simulink model "Demonstration1_2024b"  (R2024b)
settings: Solver=ode15s  StartTime=0.0  StopTime=10  RelTol=1e-4
InitFcn:
  | clear all;
  | 
  | % Bauteilgrößen
  | R = 1e3;
  | L = 10e-3;
  | C1 = 100e-9;
  | C2 = 1e-6;
  | 
  | % weitere physikalische Größen
  | k  = 1.380649e-23;
  | e  = 1.602176634e-19;
  | T_C = 25;
  | T_K = 273.15;
  | T = T_C + T_K;
  | UT = k*T/e;
  | IS = 10e-9;
  | 
  | % U0 allgemein
  | U0 = 12;
  | 
  | % I0 für Regelstrecke (1. Fall)
  | I0_1 = 1e-3;
  | 
  | % I0 für Regelstrecke (2. Fall)
  | I0_2 = 3e-3;
  | 
  | % I0 für Regelstrecke (3. Fall)
  | I0_3 = 6e-3;
  | 
  | % I0 für lineare Zustandsrückführung
  | I0_ZRF = 10e-3;
  | 
  | % Berechnung von U2 in der GGL
  | U2_bar = -UT*log(1e8*I0_ZRF);
  | 
  | % Vorgabe der Eigenwerte
  | eigenvalues_ZRF = [-2-2i; -2+2i; -10];
  | 
  | % Jacobi-Matrizen an der GGL
  | A_ZRF = [0 IS/(C1*UT)*exp(-U2_bar/UT) 1/C1;
  |      	 0 0 1/C2;
  |          -1/L -1/L -R/L];
  | B_ZRF = [0, 0;
  |          0, -1/C2;
  |          1/L, 0];
  | 
  | % Reglermatrix für lineare ZRF
  | G_ZRF = place(A_ZRF,B_ZRF,eigenvalues_ZRF);
settings Model: Creator=richa  LastModifiedBy=richa
settings ConfigComp: CovBoundaryAbsTol=1.0e-5

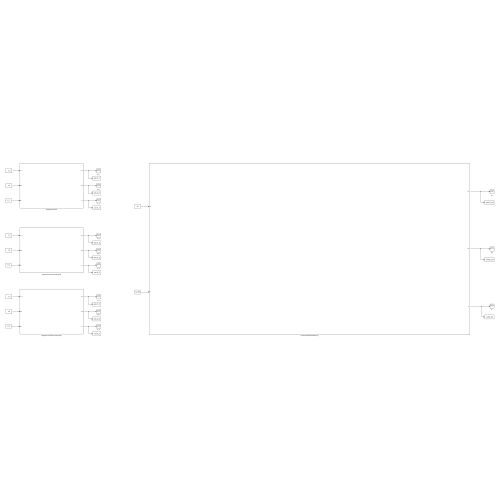
[thumbnail: Simulink's stored preview of the top-level diagram]
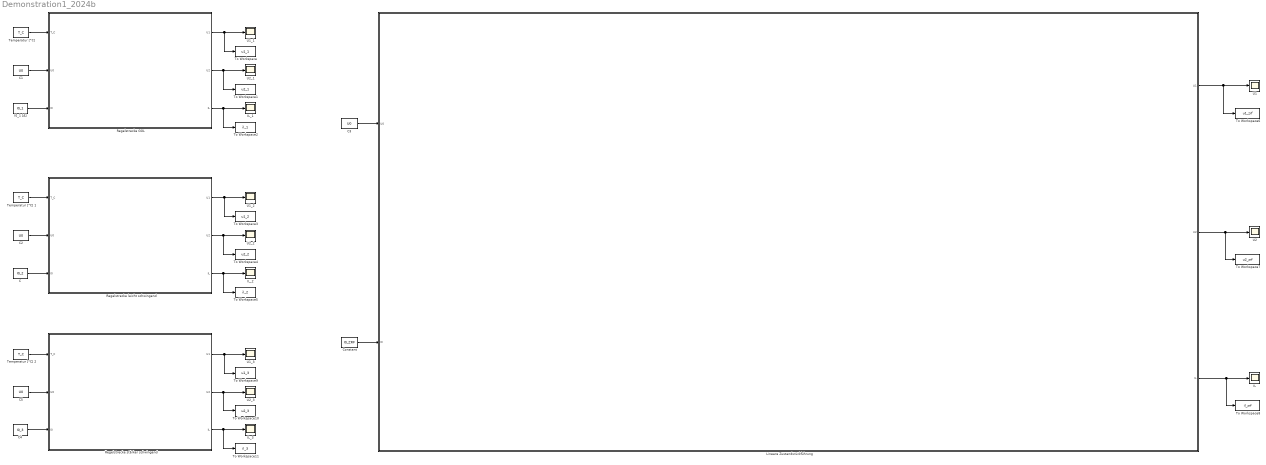
== system Demonstration1_2024b ==
  C : Constant  Value=I0_2
  C{1..3,5} (4 alike) : Constant  Value=U0
  C4 : Constant  Value=I0_3
  Constant : Constant  Value=I0_ZRF
  I0_1 [A] : Constant  Value=I0_1
  IL : Scope
  IL_1 : Scope
  IL_2 : Scope
  IL_3 : Scope
  Lineare Zustandsrückführung : Subsystem
  Regelstrecke GGL : Subsystem
  Regelstrecke leicht schwingend : Subsystem
  Regelstrecke stärker schwingend : Subsystem
  "Temperatur [°C] " : Constant  Value=T_C
  Temperatur [°C] 1 : Constant  Value=T_C
  Temperatur [°C] 2 : Constant  Value=T_C
  To Workspace : ToWorkspace  VariableName=u1_1  SaveFormat=Structure With Time  SampleTime=-1
  To Workspace1 : ToWorkspace  VariableName=u2_1  SaveFormat=Structure With Time  SampleTime=-1
  To Workspace10 : ToWorkspace  VariableName=u2_3  SaveFormat=Structure With Time  SampleTime=-1
  To Workspace11 : ToWorkspace  VariableName=il_3  SaveFormat=Structure With Time  SampleTime=-1
  To Workspace2 : ToWorkspace  VariableName=il_1  SaveFormat=Structure With Time  SampleTime=-1
  To Workspace3 : ToWorkspace  VariableName=u1_2  SaveFormat=Structure With Time  SampleTime=-1
  To Workspace4 : ToWorkspace  VariableName=u2_2  SaveFormat=Structure With Time  SampleTime=-1
  To Workspace5 : ToWorkspace  VariableName=il_2  SaveFormat=Structure With Time  SampleTime=-1
  To Workspace6 : ToWorkspace  VariableName=u1_zrf  SaveFormat=Structure With Time  SampleTime=-1
  To Workspace7 : ToWorkspace  VariableName=u2_zrf  SaveFormat=Structure With Time  SampleTime=-1
  To Workspace8 : ToWorkspace  VariableName=il_zrf  SaveFormat=Structure With Time  SampleTime=-1
  To Workspace9 : ToWorkspace  VariableName=u1_3  SaveFormat=Structure With Time  SampleTime=-1
  U1 : Scope
  U1_1 : Scope
  U1_2 : Scope
  U1_3 : Scope
  U2 : Scope
  U2_1 : Scope
  U2_2 : Scope
  U2_3 : Scope
  wires:
  "Temperatur [°C] "/1 -> Regelstrecke GGL/1(T_C)
  Regelstrecke GGL/1(U1) -> U1_1/1, To Workspace/1
  Regelstrecke GGL/2(U2) -> U2_1/1, To Workspace1/1
  Regelstrecke GGL/3(IL) -> IL_1/1, To Workspace2/1
  I0_1 [A]/1 -> Regelstrecke GGL/3(I0)
  C1/1 -> Regelstrecke GGL/2(U0)
  C/1 -> Regelstrecke leicht schwingend/3(I0)
  Regelstrecke leicht schwingend/3(IL) -> IL_2/1, To Workspace5/1
  Regelstrecke leicht schwingend/2(U2) -> U2_2/1, To Workspace4/1
  Regelstrecke leicht schwingend/1(U1) -> U1_2/1, To Workspace3/1
  Lineare Zustandsrückführung/3(IL) -> To Workspace8/1, IL/1
  Lineare Zustandsrückführung/1(U1) -> To Workspace6/1, U1/1
  Lineare Zustandsrückführung/2(U2) -> To Workspace7/1, U2/1
  Constant/1 -> Lineare Zustandsrückführung/2(I0)
  Temperatur [°C] 1/1 -> Regelstrecke leicht schwingend/1(T_C)
  C2/1 -> Regelstrecke leicht schwingend/2(U0)
  C3/1 -> Lineare Zustandsrückführung/1(U0)
  C4/1 -> Regelstrecke stärker schwingend/3(I0)
  C5/1 -> Regelstrecke stärker schwingend/2(U0)
  Regelstrecke stärker schwingend/2(U2) -> U2_3/1, To Workspace10/1
  Regelstrecke stärker schwingend/1(U1) -> U1_3/1, To Workspace9/1
  Regelstrecke stärker schwingend/3(IL) -> IL_3/1, To Workspace11/1
  Temperatur [°C] 2/1 -> Regelstrecke stärker schwingend/1(T_C)

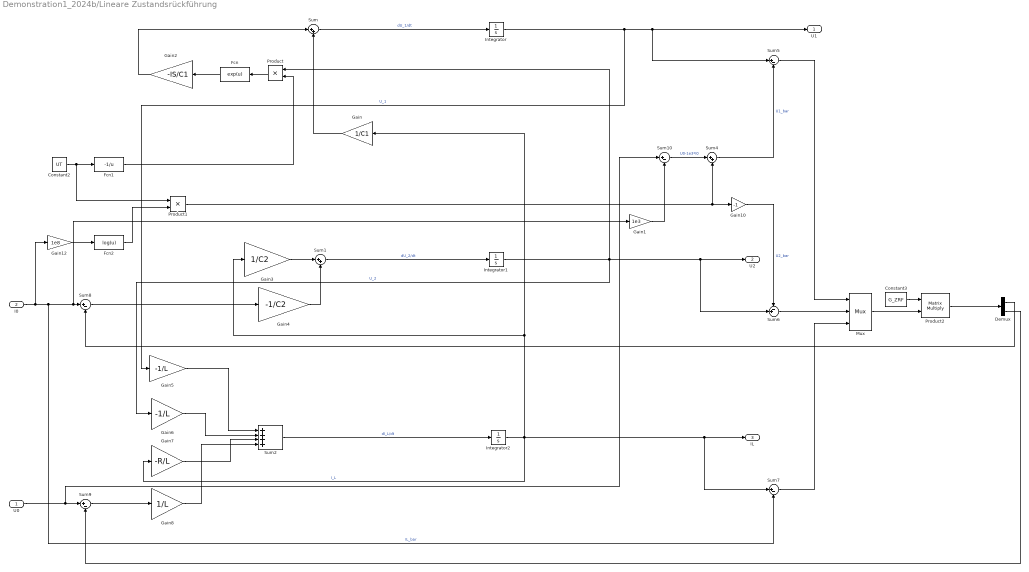
== system Demonstration1_2024b/Lineare Zustandsrückführung ==
  U0 : Inport
  I0 : Inport  Port=2
  Constant2 : Constant  Value=UT
  Constant3 : Constant  Value=G_ZRF
  Demux : Demux  Outputs=2
  Fcn : Fcn  Expr=exp(u)
  Fcn1 : Fcn  Expr=-1/u
  Fcn2 : Fcn  Expr=log(u)
  Gain : Gain  Gain=1/C1
  Gain1 : Gain  Gain=1e3
  Gain10 : Gain  Gain=-1
  Gain12 : Gain  Gain=1e8
  Gain2 : Gain  Gain=-IS/C1
  Gain3 : Gain  Gain=1/C2
  Gain4 : Gain  Gain=-1/C2
  Gain5 : Gain  Gain=-1/L
  Gain6 : Gain  Gain=-1/L
  Gain7 : Gain  Gain=-R/L
  Gain8 : Gain  Gain=1/L
  Integrator : Integrator
  Integrator1 : Integrator
  Integrator2 : Integrator
  Mux : Mux  Inputs=3
  Product : Product
  Product1 : Product
  Product2 : Product  Multiplication=Matrix(*)
  Sum : Sum  Inputs=|++
  Sum1 : Sum  Inputs=|++
  Sum{5,7..10} (5 alike) : Sum  Inputs=|+-
  Sum2 : Sum  Inputs=++++
  Sum4 : Sum  Inputs=|++
  Sum6 : Sum  Inputs=-+|
  U1 : Outport
  U2 : Outport  Port=2
  IL : Outport  Port=3
  wires:
  Integrator/1 -> U1/1, Sum5/1, Gain5/1  "U_1"
  Integrator2/1 -> Gain/1, Gain3/1, Gain7/1, IL/1, Sum7/1  "I_L"
  Gain4/1 -> Sum1/2
  Product/1 -> Fcn/1
  Constant2/1 -> Product1/1, Fcn1/1
  Gain/1 -> Sum/2
  Integrator1/1 -> U2/1, Sum6/2, Product/1, Gain6/1  "U_2"
  Gain10/1 -> Sum6/1  "U2_bar"
  Gain8/1 -> Sum2/4
  Gain3/1 -> Sum1/1
  I0/1 -> Gain12/1, Gain1/1, Sum8/1, Sum7/2  "IL_bar"
  Sum/1 -> Integrator/1  "dU_1/dt"
  Sum5/1 -> Mux/1
  Fcn1/1 -> Product/2
  Sum6/1 -> Mux/2
  Demux/2 -> Sum9/2
  Gain2/1 -> Sum/1
  Gain5/1 -> Sum2/1
  Sum8/1 -> Gain4/1
  Sum2/1 -> Integrator2/1  "dI_L/dt"
  Gain6/1 -> Sum2/2
  Sum4/1 -> Sum5/2  "U1_bar"
  Mux/1 -> Product2/2
  Sum10/1 -> Sum4/1  "U0-1e3*I0"
  Sum9/1 -> Gain8/1
  Product1/1 -> Gain10/1, Sum4/2
  Demux/1 -> Sum8/2
  Gain7/1 -> Sum2/3
  Fcn/1 -> Gain2/1
  Sum1/1 -> Integrator1/1  "dU_2/dt"
  Sum7/1 -> Mux/3
  Gain12/1 -> Fcn2/1
  Fcn2/1 -> Product1/2
  Gain1/1 -> Sum10/2
  Product2/1 -> Demux/1
  Constant3/1 -> Product2/1
  U0/1 -> Sum9/1, Sum10/1

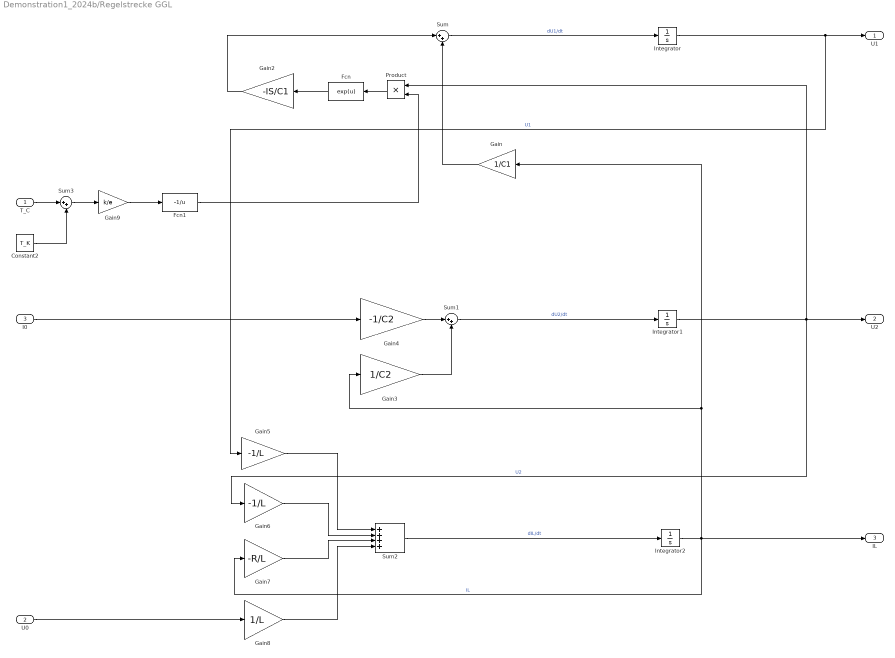
== system Demonstration1_2024b/Regelstrecke GGL ==
  T_C : Inport
  U0 : Inport  Port=2
  I0 : Inport  Port=3
  Constant2 : Constant  Value=T_K
  Fcn : Fcn  Expr=exp(u)
  Fcn1 : Fcn  Expr=-1/u
  Gain : Gain  Gain=1/C1
  Gain2 : Gain  Gain=-IS/C1
  Gain3 : Gain  Gain=1/C2
  Gain4 : Gain  Gain=-1/C2
  Gain5 : Gain  Gain=-1/L
  Gain6 : Gain  Gain=-1/L
  Gain7 : Gain  Gain=-R/L
  Gain8 : Gain  Gain=1/L
  Gain9 : Gain  Gain=k/e
  Integrator : Integrator
  Integrator1 : Integrator
  Integrator2 : Integrator
  Product : Product
  Sum : Sum  Inputs=|++
  Sum1 : Sum  Inputs=|++
  Sum2 : Sum  Inputs=++++
  Sum3 : Sum  Inputs=|++
  U1 : Outport
  U2 : Outport  Port=2
  IL : Outport  Port=3
  wires:
  Sum/1 -> Integrator/1  "dU1/dt"
  Integrator/1 -> U1/1, Gain5/1  "U1"
  Sum3/1 -> Gain9/1
  Gain2/1 -> Sum/1
  Gain8/1 -> Sum2/4
  Fcn1/1 -> Product/2
  Gain/1 -> Sum/2
  Gain9/1 -> Fcn1/1
  Gain5/1 -> Sum2/1
  I0/1 -> Gain4/1
  Gain7/1 -> Sum2/3
  U0/1 -> Gain8/1
  Sum1/1 -> Integrator1/1  "dU2/dt"
  Gain6/1 -> Sum2/2
  Integrator2/1 -> IL/1, Gain3/1, Gain/1, Gain7/1  "IL"
  Sum2/1 -> Integrator2/1  "dIL/dt"
  Gain4/1 -> Sum1/1
  Integrator1/1 -> U2/1, Product/1, Gain6/1  "U2"
  Constant2/1 -> Sum3/2
  Product/1 -> Fcn/1
  Fcn/1 -> Gain2/1
  Gain3/1 -> Sum1/2
  T_C/1 -> Sum3/1

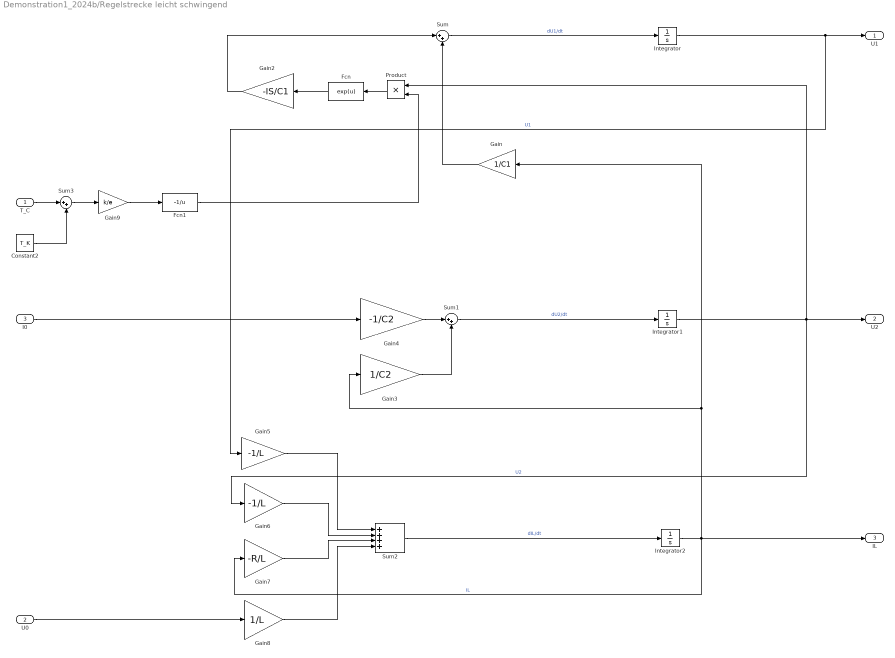
== system Demonstration1_2024b/Regelstrecke leicht schwingend ==
  T_C : Inport
  U0 : Inport  Port=2
  I0 : Inport  Port=3
  Constant2 : Constant  Value=T_K
  Fcn : Fcn  Expr=exp(u)
  Fcn1 : Fcn  Expr=-1/u
  Gain : Gain  Gain=1/C1
  Gain2 : Gain  Gain=-IS/C1
  Gain3 : Gain  Gain=1/C2
  Gain4 : Gain  Gain=-1/C2
  Gain5 : Gain  Gain=-1/L
  Gain6 : Gain  Gain=-1/L
  Gain7 : Gain  Gain=-R/L
  Gain8 : Gain  Gain=1/L
  Gain9 : Gain  Gain=k/e
  Integrator : Integrator
  Integrator1 : Integrator
  Integrator2 : Integrator
  Product : Product
  Sum : Sum  Inputs=|++
  Sum1 : Sum  Inputs=|++
  Sum2 : Sum  Inputs=++++
  Sum3 : Sum  Inputs=|++
  U1 : Outport
  U2 : Outport  Port=2
  IL : Outport  Port=3
  wires:
  Sum/1 -> Integrator/1  "dU1/dt"
  Integrator/1 -> U1/1, Gain5/1  "U1"
  Sum3/1 -> Gain9/1
  Gain2/1 -> Sum/1
  Gain8/1 -> Sum2/4
  Fcn1/1 -> Product/2
  Gain/1 -> Sum/2
  Gain9/1 -> Fcn1/1
  Gain5/1 -> Sum2/1
  I0/1 -> Gain4/1
  Gain7/1 -> Sum2/3
  U0/1 -> Gain8/1
  Sum1/1 -> Integrator1/1  "dU2/dt"
  Gain6/1 -> Sum2/2
  Integrator2/1 -> IL/1, Gain3/1, Gain/1, Gain7/1  "IL"
  Sum2/1 -> Integrator2/1  "dIL/dt"
  Gain4/1 -> Sum1/1
  Integrator1/1 -> U2/1, Product/1, Gain6/1  "U2"
  Constant2/1 -> Sum3/2
  Product/1 -> Fcn/1
  Fcn/1 -> Gain2/1
  Gain3/1 -> Sum1/2
  T_C/1 -> Sum3/1

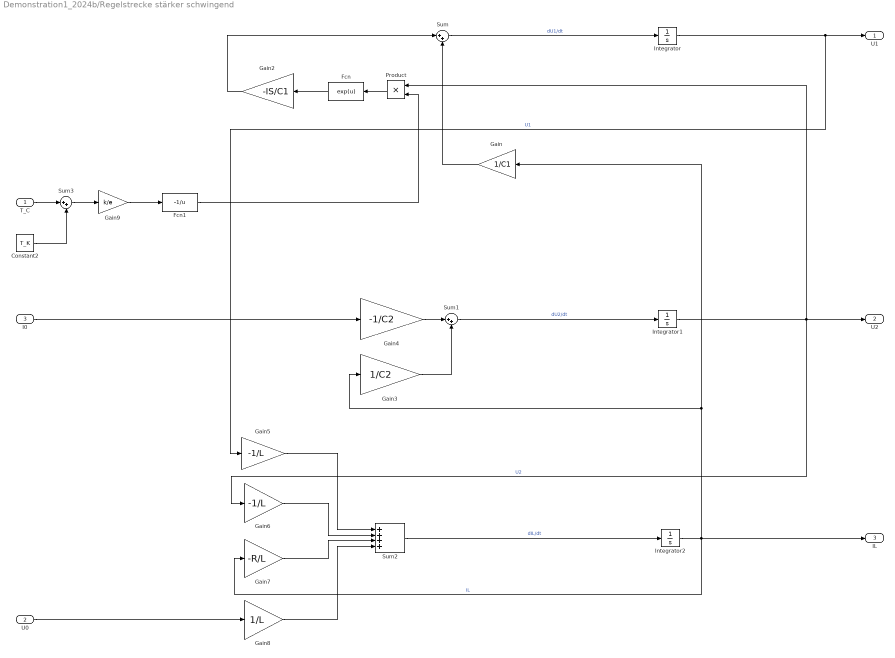
== system Demonstration1_2024b/Regelstrecke stärker schwingend ==
  T_C : Inport
  U0 : Inport  Port=2
  I0 : Inport  Port=3
  Constant2 : Constant  Value=T_K
  Fcn : Fcn  Expr=exp(u)
  Fcn1 : Fcn  Expr=-1/u
  Gain : Gain  Gain=1/C1
  Gain2 : Gain  Gain=-IS/C1
  Gain3 : Gain  Gain=1/C2
  Gain4 : Gain  Gain=-1/C2
  Gain5 : Gain  Gain=-1/L
  Gain6 : Gain  Gain=-1/L
  Gain7 : Gain  Gain=-R/L
  Gain8 : Gain  Gain=1/L
  Gain9 : Gain  Gain=k/e
  Integrator : Integrator
  Integrator1 : Integrator
  Integrator2 : Integrator
  Product : Product
  Sum : Sum  Inputs=|++
  Sum1 : Sum  Inputs=|++
  Sum2 : Sum  Inputs=++++
  Sum3 : Sum  Inputs=|++
  U1 : Outport
  U2 : Outport  Port=2
  IL : Outport  Port=3
  wires:
  Sum/1 -> Integrator/1  "dU1/dt"
  Integrator/1 -> U1/1, Gain5/1  "U1"
  Sum3/1 -> Gain9/1
  Gain2/1 -> Sum/1
  Gain8/1 -> Sum2/4
  Fcn1/1 -> Product/2
  Gain/1 -> Sum/2
  Gain9/1 -> Fcn1/1
  Gain5/1 -> Sum2/1
  I0/1 -> Gain4/1
  Gain7/1 -> Sum2/3
  U0/1 -> Gain8/1
  Sum1/1 -> Integrator1/1  "dU2/dt"
  Gain6/1 -> Sum2/2
  Integrator2/1 -> IL/1, Gain3/1, Gain/1, Gain7/1  "IL"
  Sum2/1 -> Integrator2/1  "dIL/dt"
  Gain4/1 -> Sum1/1
  Integrator1/1 -> U2/1, Product/1, Gain6/1  "U2"
  Constant2/1 -> Sum3/2
  Product/1 -> Fcn/1
  Fcn/1 -> Gain2/1
  Gain3/1 -> Sum1/2
  T_C/1 -> Sum3/1
